simulink model "microgrid_slg"  (R2025b)
settings: Solver=FixedStepAuto  StartTime=0.0  StopTime=1  RelTol=1e-3
settings Model: Creator=User  LastModifiedBy=User

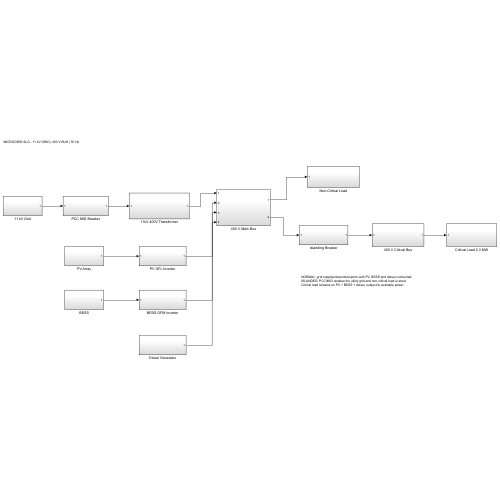
[thumbnail: Simulink's stored preview of the top-level diagram]
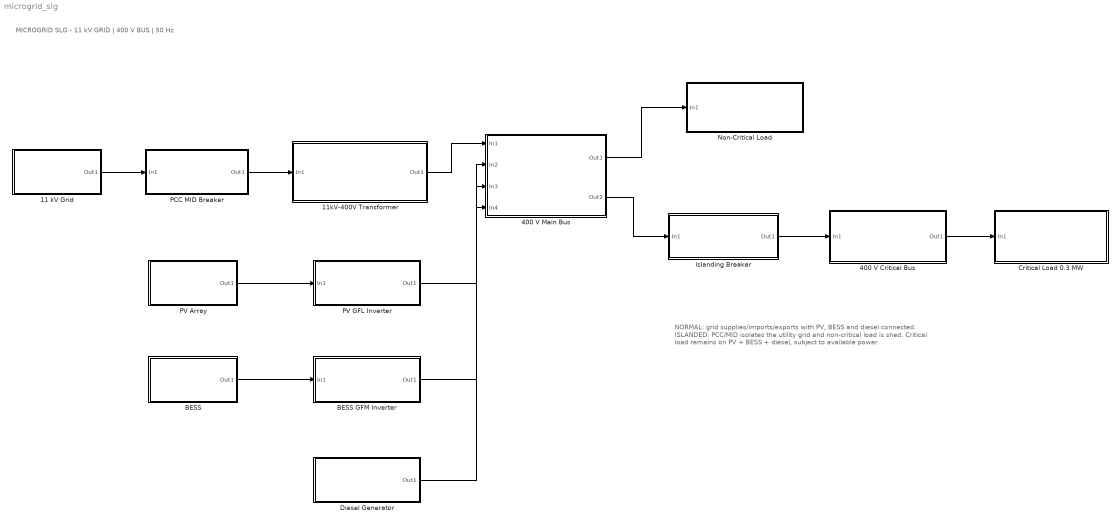
== system microgrid_slg ==
  note: MICROGRID SLG - 11 kV GRID | 400 V BUS | 50 Hz
  note: NORMAL: grid supplies/imports/exports with PV, BESS and diesel connected.
      | ISLANDED: PCC/MID isolates the utility grid and non-critical load is shed.
      | Critical load remains on PV + BESS + diesel, subject to available power.
  11 kV Grid : Subsystem
  11kV-400V Transformer : Subsystem
  400 V Critical Bus : Subsystem
  400 V Main Bus : Subsystem
  BESS : Subsystem
  BESS GFM Inverter : Subsystem
  Critical Load 0.3 MW : Subsystem
  Diesel Generator : Subsystem
  Islanding Breaker : Subsystem
  Non-Critical Load : Subsystem
  PCC MID Breaker : Subsystem
  PV Array : Subsystem
  PV GFL Inverter : Subsystem
  wires:
  11 kV Grid/1(Out1) -> PCC MID Breaker/1(In1)
  PCC MID Breaker/1(Out1) -> 11kV-400V Transformer/1(In1)
  11kV-400V Transformer/1(Out1) -> 400 V Main Bus/1(In1)
  PV Array/1(Out1) -> PV GFL Inverter/1(In1)
  PV GFL Inverter/1(Out1) -> 400 V Main Bus/2(In2)
  BESS/1(Out1) -> BESS GFM Inverter/1(In1)
  BESS GFM Inverter/1(Out1) -> 400 V Main Bus/3(In3)
  Diesel Generator/1(Out1) -> 400 V Main Bus/4(In4)
  400 V Main Bus/1(Out1) -> Non-Critical Load/1(In1)
  400 V Main Bus/2(Out2) -> Islanding Breaker/1(In1)
  Islanding Breaker/1(Out1) -> 400 V Critical Bus/1(In1)
  400 V Critical Bus/1(Out1) -> Critical Load 0.3 MW/1(In1)

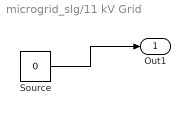
== system microgrid_slg/11 kV Grid ==
  Source : Constant  Value=0
  Out1 : Outport
  wires:
  Source/1 -> Out1/1

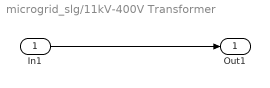
== system microgrid_slg/11kV-400V Transformer ==
  In1 : Inport
  Out1 : Outport
  wires:
  In1/1 -> Out1/1

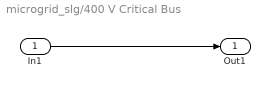
== system microgrid_slg/400 V Critical Bus ==
  In1 : Inport
  Out1 : Outport
  wires:
  In1/1 -> Out1/1

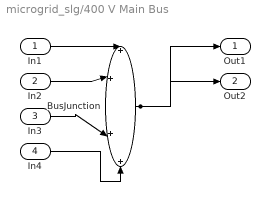
== system microgrid_slg/400 V Main Bus ==
  In1 : Inport
  In2 : Inport  Port=2
  In3 : Inport  Port=3
  In4 : Inport  Port=4
  BusJunction : Sum  Inputs=++++
  Out1 : Outport
  Out2 : Outport  Port=2
  wires:
  In1/1 -> BusJunction/1
  In2/1 -> BusJunction/2
  In3/1 -> BusJunction/3
  In4/1 -> BusJunction/4
  BusJunction/1 -> Out1/1, Out2/1

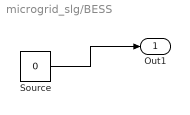
== system microgrid_slg/BESS ==
  Source : Constant  Value=0
  Out1 : Outport
  wires:
  Source/1 -> Out1/1

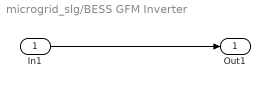
== system microgrid_slg/BESS GFM Inverter ==
  In1 : Inport
  Out1 : Outport
  wires:
  In1/1 -> Out1/1

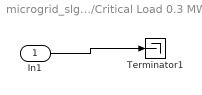
== system microgrid_slg/Critical Load 0.3 MW ==
  In1 : Inport
  Terminator1 : Terminator
  wires:
  In1/1 -> Terminator1/1

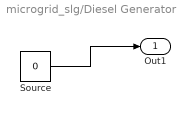
== system microgrid_slg/Diesel Generator ==
  Source : Constant  Value=0
  Out1 : Outport
  wires:
  Source/1 -> Out1/1

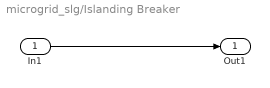
== system microgrid_slg/Islanding Breaker ==
  In1 : Inport
  Out1 : Outport
  wires:
  In1/1 -> Out1/1

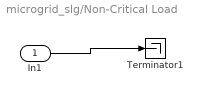
== system microgrid_slg/Non-Critical Load ==
  In1 : Inport
  Terminator1 : Terminator
  wires:
  In1/1 -> Terminator1/1

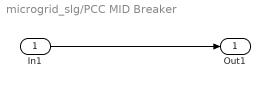
== system microgrid_slg/PCC MID Breaker ==
  In1 : Inport
  Out1 : Outport
  wires:
  In1/1 -> Out1/1

== system microgrid_slg/PV Array ==
  Source : Constant  Value=0
  Out1 : Outport
  wires:
  Source/1 -> Out1/1

== system microgrid_slg/PV GFL Inverter ==
  In1 : Inport
  Out1 : Outport
  wires:
  In1/1 -> Out1/1
